simulink model "a01_01simulink"  (R2022a)
settings: Solver=VariableStepAuto  StartTime=0.0  StopTime=10.0  RelTol=1e-3
settings Model: Creator=Waine  LastModifiedBy=Waine

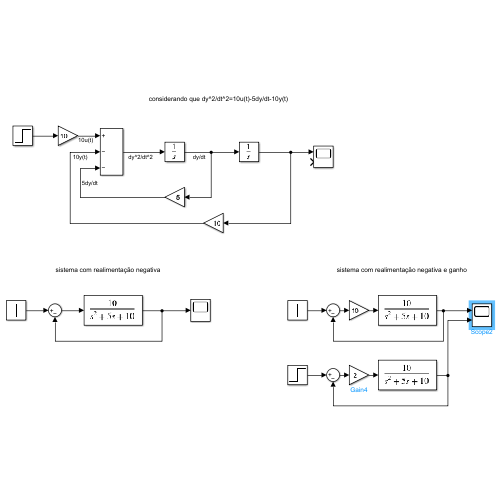
[thumbnail: Simulink's stored preview of the top-level diagram]
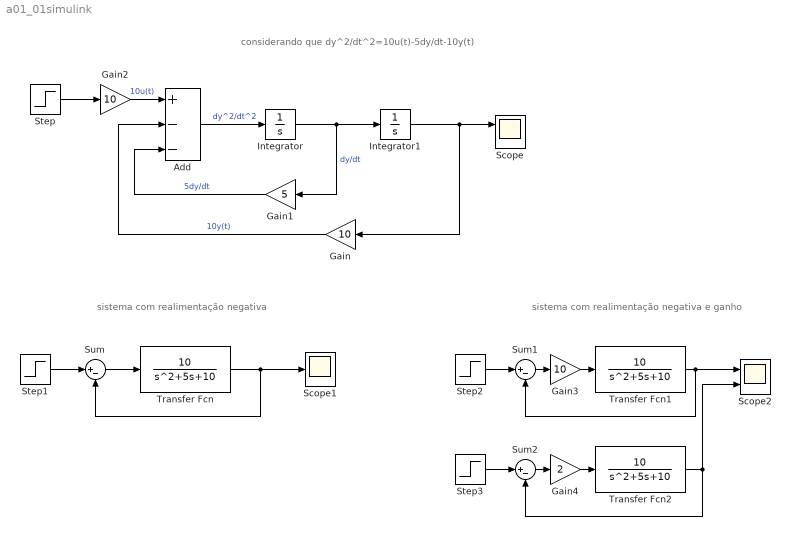
== system a01_01simulink ==
  note: sistema com realimentação negativa
  note: considerando que dy^2/dt^2=10u(t)-5dy/dt-10y(t)
  note: sistema com realimentação negativa e ganho
  Add : Sum  Inputs=+--
  Gain : Gain  Gain=10
  Gain1 : Gain  Gain=5
  Gain2 : Gain  Gain=10
  Gain3 : Gain  Gain=10
  Gain4 : Gain  Gain=2
  Integrator : Integrator
  Integrator1 : Integrator
  Scope : Scope  NumInputPorts=2
  Scope1 : Scope
  Scope2 : Scope  NumInputPorts=2
  Step{,1..3} (4 alike) : Step  SampleTime=0
  Sum : Sum  Inputs=|+-
  Sum1 : Sum  Inputs=|+-
  Sum2 : Sum  Inputs=|+-
  Transfer Fcn : TransferFcn  Numerator=[10]  Denominator=[1 5 10]
  Transfer Fcn1 : TransferFcn  Numerator=[10]  Denominator=[1 5 10]
  Transfer Fcn2 : TransferFcn  Numerator=[10]  Denominator=[1 5 10]
  wires:
  Gain/1 -> Add/2  "10y(t)"
  Gain1/1 -> Add/3  "5dy/dt"
  Add/1 -> Integrator/1  "dy^2/dt^2"
  Integrator/1 -> Gain1/1, Integrator1/1  "dy/dt"
  Integrator1/1 -> Scope/1, Gain/1
  Step/1 -> Gain2/1
  Gain2/1 -> Add/1  "10u(t)"
  Transfer Fcn/1 -> Sum/2, Scope1/1
  Step1/1 -> Sum/1
  Sum/1 -> Transfer Fcn/1
  Transfer Fcn1/1 -> Sum1/2, Scope2/1
  Step2/1 -> Sum1/1
  Sum1/1 -> Gain3/1
  Gain3/1 -> Transfer Fcn1/1
  Sum2/1 -> Gain4/1
  Step3/1 -> Sum2/1
  Gain4/1 -> Transfer Fcn2/1
  Transfer Fcn2/1 -> Scope2/2, Sum2/2
